simulink model "simpletontester"  (R2014b)
settings: Solver=ode45  StartTime=0.0  StopTime=1000.0  RelTol=1e-3
values from neighbouring files (symbols this model uses):
  a0 = ((Rt1*cs1*cs2+cs1*(Rt2*cs2+cs1*(Rt2*cs2+Rt3*cs2))))/(cs1*cs2)    (= 5000100)    [przypadkowy_kod.m]
  a1 = ((I1*cs1*cs2+Rt1*(Rt3*cs1+Rt2*cs2+Rt3*cs2)+cs1*(Rt1+Rt2+I3*cs2+I3*cs2+I2*cs2+I3*cs1)))/(cs1*cs2)    (= 5.152)    [przypadkowy_kod.m]    (also in zmiennefuruta.m = 0)
  a2 = (I1*(Rt3*cs1+Rt2*cs2+Rt3*cs2)+Rt1*(Rt2*Rt3+I3*cs2+I2*cs2+I3*cs1)+cs1*(I2*Rt3+I3*Rt2))/(cs1*cs2)    (= 0.00805)    [przypadkowy_kod.m]    (also in zmiennefuruta.m = -44.5909090909)
  a3 = ((I1*(Rt2*Rt3+I3*cs2+I2*cs2+I3*cs1)+Rt1*(I2*Rt3+I3*Rt2)+cs1*I2*I3))/(cs1*cs2)    (= 8.3e-05)    [przypadkowy_kod.m]    (also in zmiennefuruta.m = 4.41818181818)
  I1 = 1    [przypadkowy_kod.m]    (also in ssssss.m; vars.m = 20)
  Rt1 = 50    [przypadkowy_kod.m]    (also in ssssss.m = 10; vars.m = 1)
settings Model: Creator=Jacek  LastModifiedBy=Jacek

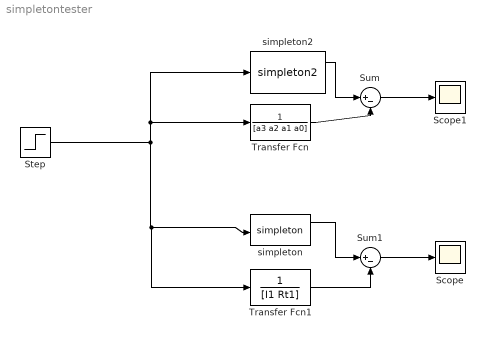
== system simpletontester ==
  Scope : Scope
  Scope1 : Scope
  Step : Step  Time=0  After=1000  SampleTime=0
  Sum : Sum  Inputs=|+-
  Sum1 : Sum  Inputs=|+-
  Transfer Fcn : TransferFcn  Denominator=[a3 a2 a1 a0]
  Transfer Fcn1 : TransferFcn  Denominator=[I1 Rt1]
  simpleton : S-Function  FunctionName=simpleton  EnableBusSupport=off
      mask Display: port_label('input',1,'Input_Interface_Component.'); port_label('output',1,'Output_Interface_Component.'); port_label('output',2,'DEBUG')
  simpleton2 : S-Function  FunctionName=simpleton2  EnableBusSupport=off
      mask Display: port_label('input',1,'Input_Interface_Component.'); port_label('output',1,'Output_Interface_Component.'); port_label('output',2,'DEBUG')
  wires:
  Step/1 -> Transfer Fcn1/1, simpleton/1, Transfer Fcn/1, simpleton2/1
  Sum/1 -> Scope1/1
  simpleton2/1 -> Sum/1
  Transfer Fcn/1 -> Sum/2
  simpleton/1 -> Sum1/1
  Transfer Fcn1/1 -> Sum1/2
  Sum1/1 -> Scope/1
